simulink model "EF"  (R2023a)
settings: Solver=FixedStepDiscrete  StartTime=0.0  StopTime=inf  FixedStep=50e-6  RelTol=1e-3  EnableMultiTasking=on
libraries: spsThreePhaseFaultLib x11, spsThreePhaseSourceLib x3, spsCurrentMeasurementLib x2, spsDistributedParametersLineLib x2, spsGroundLib x2, spsThreePhaseParallelRLCLoadLib x2, spsThreePhaseTransformer12TerminalsLib x2, spsThreePhaseSeriesRLCLoadLib x1, spsThreePhaseVIMeasurementLib x1, instrumentlib x1, spspowerguiLib x1
settings Model: Creator=Administrator  LastModifiedBy=Ansoufeh
settings SolverCC: AlgebraicLoopSolver=TrustRegion
settings DataIOCC: LimitDataPoints=on  SaveFormat=Array  SignalLoggingSaveFormat=ModelDataLogs  ReturnWorkspaceOutputs=off
settings OptimizationCC: ExpressionDepthLimit=2147483647  LifeSpan=inf
settings DebuggingCC: UnderspecifiedInitializationDetection=Classic  MergeDetectMultiDrivingBlocksExec=none  SolverPrmCheckMsg=warning  FcnCallInpInsideContextMsg=warning  StateNameClashWarn=warning  SFUnexpectedBacktrackingDiag=warning  SFNoUnconditionalDefaultTransitionDiag=warning  SFExecutionAtInitializationDiag=none  ArithmeticOperatorsInVariantConditions=warning
settings HardwareCC: ProdBitPerPointer=32  ProdBitPerSizeT=32  ProdBitPerPtrDiffT=32  ProdLargestAtomicFloat=None  ProdIntDivRoundTo=Undefined  ProdEndianess=Unspecified  ProdWordSize=32  ProdHWDeviceType=32-bit Generic
settings ModelReferenceCC: EnableRefExpFcnMdlSchedulingChecks=on  PropagateSignalLabelsOutOfModel=off
settings SFSimCC: SimUseLocalCustomCode=off  CustomCodeUndefinedFunction=UseInterfaceOnly
settings RTWCC: RTWUseLocalCustomCode=off
settings CodeAppCC: StateflowObjectComments=on
settings GRTTargetCC: TargetLangStandard=C89/C90 (ANSI)  CombineOutputUpdateFcns=off  GRTInterface=on
settings ConfigComp: CovMetricSettings=dw  CovSaveCumulativeToWorkspaceVar=on  CovSaveSingleToWorkspaceVar=on  CovExternalEMLEnable=off  CovSFcnEnable=off
settings SimscapeCC: SimscapeNormalizeSystem=off

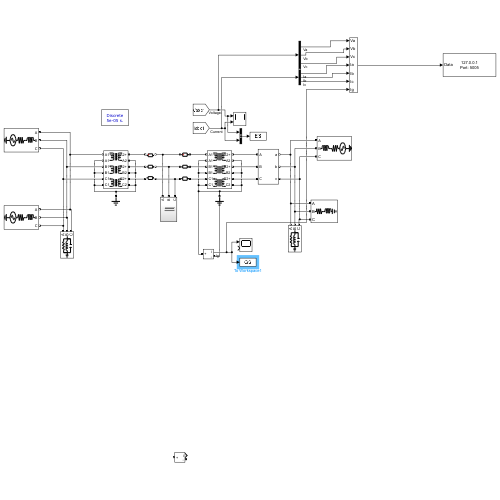
[thumbnail: Simulink's stored preview of the top-level diagram]
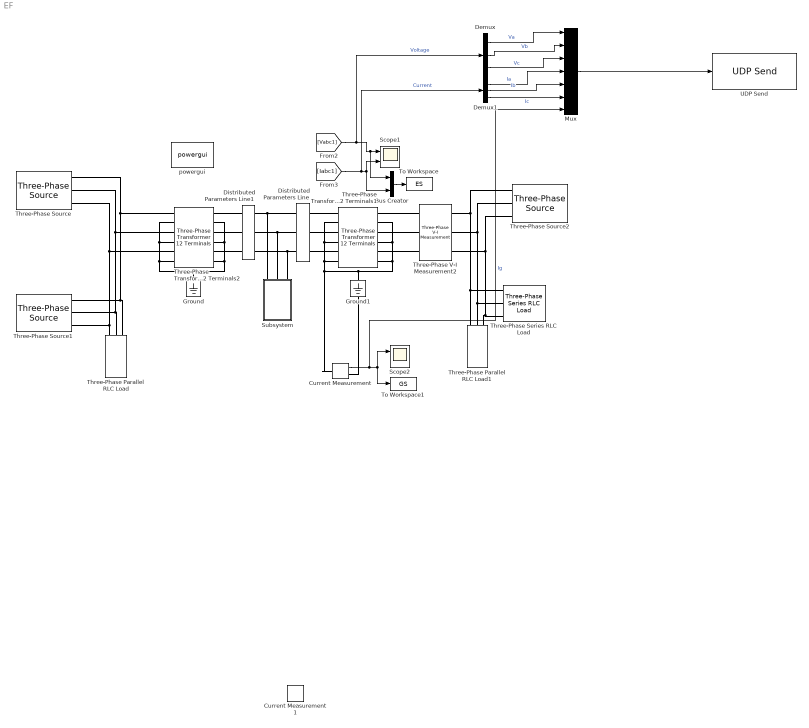
== system EF ==
  Bus Creator : BusCreator  Inputs=2
  Current Measurement : spsCurrentMeasurementLib/Current Measurement  PhasorSimulation=off  OutputType=Complex  PSBequivalent=0
  Current Measurement1 : spsCurrentMeasurementLib/Current Measurement  PhasorSimulation=off  OutputType=Complex  PSBequivalent=0
  Demux : Demux  Outputs=3
  Demux1 : Demux  Outputs=3
  Distributed Parameters Line : spsDistributedParametersLineLib/Distributed Parameters Line  Phases=3  Length=33  Frequency=50  Resistance=[0.0132 0.132]  Inductance="[0.9337e-3  4.1264e-3]"  Capacitance=[12.74e-9 7.751e-9]  x1=[-0.0002 -26194.4990565152 0 0;-0.00015 -25142.4200654069 -14084.2021249757 -139676.156535357;-0.0001 -24084.1375583615 -10869.3978359019 -138608.787184405;-5e-05 -23019.9126507524 -7651.91168555439 -137507.218189264]  x2=[-0.0002 -26508.8832650109 0 0;-0.00015 -25460.9682547841 -14346.2347519264 -139705.26954599;-0.0001 -24406.7711316212 -11133.032561043 -138641.209662973;-5e-05 -23346.5520028879 -7917.08346096219 -137542.942136005]  x3=[-0.0002 -32.9787723954412 0 0;-0.00015 -31.6839639948928 -55.9550231746791 -498.136583373614;-0.0001 -30.3813380503261 -44.5400586108173 -494.408000929939;-5e-05 -29.0712159652011 -33.1141044539605 -490.557430710021]  x4=[-0.0002 -44.2714402477354 0 0;-0.00015 -42.7334839975939 -75.9286566808512 -541.426288335773;-0.0001 -41.1849838997108 -63.6542106681894 -537.579668417394;-5e-05 -39.6263220233146 -51.3640589315235 -533.600408759809]  x5=0.000186628717108595  V1=[2.547e-09 1.32e+05 1.32e+05;314.2 314.2 314.2;-0.1043 0.8095 -0.7613]  V2=[2.522e-09 1.32e+05 1.32e+05;314.2 314.2 314.2;-0.1193 0.8007 -0.7701]  I1=[2.615e-12 367.2 367.2;314.2 314.2 314.2;-0.5343 0.7771 -0.7937]  I2=[5.144e-12 607 607;314.2 314.2 314.2;-0.488 0.7934 -0.7774]  nHarmo=1  Measurements=None  Decoupling=off  VsMag0=0  VrMag0=0  VsAngle0=0  VrAngle0=0  IsMag0=0  IrMag0=0  IsAngle0=0  IrAngle0=0
      settings: LibrarySourceBlock=sps_lib/Power Grid Elements/Distributed Parameters Line
  Distributed Parameters Line1 : spsDistributedParametersLineLib/Distributed Parameters Line  Phases=3  Length=33  Frequency=50  Resistance=[0.0132 0.132]  Inductance="[0.9337e-3  4.1264e-3]"  Capacitance=[12.74e-9 7.751e-9]  x1=[-0.0002 -25744.8060541232 0 0;-0.00015 -24691.8631075608 -13770.6890303449 -139458.191007;-0.0001 -23632.8278132488 -10558.3448334587 -138388.513170059;-5e-05 -22567.9614722995 -7343.39552297271 -137284.690038246]  x2=[-0.0002 -26194.4990565152 0 0;-0.00015 -25142.4200654069 -14084.2021249757 -139676.156535357;-0.0001 -24084.1375583615 -10869.3978359019 -138608.787184405;-5e-05 -23019.9126507524 -7651.91168555439 -137507.218189264]  x3=[-0.0002 -37.5098312649845 0 0;-0.00015 -36.2542690466918 -81.6323668107199 -504.631077447372;-0.0001 -34.989761629996 -70.2873602270549 -501.193965481607;-5e-05 -33.7166210131811 -58.9250112889862 -497.633191404385]  x4=[-0.0002 -38.7109249659307 0 0;-0.00015 -37.1263797926598 -48.124582446735 -534.043951803313;-0.0001 -35.5326742407089 -35.7827477551342 -529.884875428009;-5e-05 -33.930201533076 -23.4320842059535 -525.595057888531]  x5=0.000186628717108595  V1=[2.618e-09 1.319e+05 1.319e+05;314.2 314.2 314.2;-0.1003 0.8184 -0.7524]  V2=[2.549e-09 1.32e+05 1.32e+05;314.2 314.2 314.2;-0.1043 0.8095 -0.7613]  I1=[2.387e-12 367.3 367.3;314.2 314.2 314.2;0.1434 0.7414 -0.8294]  I2=[6.175e-12 607.4 607.4;314.2 314.2 314.2;-0.4569 0.8292 -0.7416]  nHarmo=1  Measurements=None  Decoupling=off  VsMag0=0  VrMag0=0  VsAngle0=0  VrAngle0=0  IsMag0=0  IrMag0=0  IsAngle0=0  IrAngle0=0
      settings: LibrarySourceBlock=sps_lib/Power Grid Elements/Distributed Parameters Line
  Ground : spsGroundLib/Ground  LConnTagsString=a
  Ground1 : spsGroundLib/Ground  LConnTagsString=a
  Mux : Mux  Inputs=7
      settings: DisplayOption=signals
  Scope1 : Scope  NumInputPorts=2
  Scope2 : Scope  NumInputPorts=2
  Subsystem : Subsystem
  Three-Phase Parallel RLC Load : spsThreePhaseParallelRLCLoadLib/Three-Phase Parallel RLC Load  LConnTagsString=A|B|C  Configuration=Y (grounded)  NominalVoltage=1000  Vabc=[1e3 1e3 1e3]  Vabcp=[1e3 1e3 1e3]  NominalFrequency=60  UnbalancedPower=off  ActivePower=10e4  InductivePower=100  CapacitivePower=100  Pabc=[10e3 9e3 11e3]  QLabc=[100 90 110]  QCabc=[100 90 110]  Pabcp=[10e3 9e3 11e3]  QLabcp=[100 90 110]  QCabcp=[100 90 110]  Measurements=None  LoadType=constant Z
  Three-Phase Parallel RLC Load1 : spsThreePhaseParallelRLCLoadLib/Three-Phase Parallel RLC Load  LConnTagsString=A|B|C  Configuration=Y (grounded)  NominalVoltage=1000  Vabc=[1e3 1e3 1e3]  Vabcp=[1e3 1e3 1e3]  NominalFrequency=60  UnbalancedPower=off  ActivePower=100  InductivePower=10  CapacitivePower=10  Pabc=[10e3 9e3 11e3]  QLabc=[100 90 110]  QCabc=[100 90 110]  Pabcp=[10e3 9e3 11e3]  QLabcp=[100 90 110]  QCabcp=[100 90 110]  Measurements=None  LoadType=constant Z
  Three-Phase Series RLC Load : spsThreePhaseSeriesRLCLoadLib/Three-Phase Series RLC Load  LConnTagsString=A|B|C  Configuration=Y (grounded)  NominalVoltage=11e3  Vabc=[1e3 1e3 1e3]  Vabcp=[1e3 1e3 1e3]  NominalFrequency=50  UnbalancedPower=off  ActivePower=10e6  InductivePower=100  CapacitivePower=0  Pabc=[10e3 9e3 11e3]  QLabc=[100 90 110]  QCabc=[100 90 110]  Pabcp=[10e3 9e3 11e3]  QLabcp=[100 90 110]  QCabcp=[100 90 110]  Measurements=None  LoadType=constant Z
  Three-Phase V-I Measurement2 : spsThreePhaseVIMeasurementLib/Three-Phase V-I Measurement  VoltageMeasurement=phase-to-phase  SetLabelV=on  LabelV=Vabc1  Vpu=off  VpuLL=on  CurrentMeasurement=yes  SetLabelI=on  LabelI=Iabc1  Ipu=off  Pbase=100e6  Vbase=11e3  OutputType=Complex  PhasorSimulation=off  PSBequivalent=0
  Three-Phase Source : spsThreePhaseSourceLib/Three-Phase Source  InternalConnection=Yg  VoltagePhases=on  Voltage=11e3  PhaseAngle=0  Voltage_phases=[25e3 11e3 11e3]/sqrt(3)  PhaseAngles_phases=[0 -120 +120]  Frequency=50  NonIdealSource=on  SpecifyImpedance=off  Resistance=1.5  Inductance=16.58e-3  ShortCircuitLevel=50e6  BaseVoltage=11e3  XRratio=7  BusType=PV  Pref=50e6  Qref=0  Prefabc=[10e3, 10e3, 10e3]  Qrefabc=[0, 0, 0]  Qmin=-inf  Qmax=inf
  Three-Phase Source1 : spsThreePhaseSourceLib/Three-Phase Source  InternalConnection=Yg  VoltagePhases=on  Voltage=11e3  PhaseAngle=0  Voltage_phases=[25e3 11e3 11e3]/sqrt(3)  PhaseAngles_phases=[0 -120 +120]  Frequency=50  NonIdealSource=on  SpecifyImpedance=off  Resistance=1.5  Inductance=16.58e-3  ShortCircuitLevel=50e6  BaseVoltage=11e3  XRratio=7  BusType=PV  Pref=50e6  Qref=0  Prefabc=[10e3, 10e3, 10e3]  Qrefabc=[0, 0, 0]  Qmin=-inf  Qmax=inf
  Three-Phase Source2 : spsThreePhaseSourceLib/Three-Phase Source  InternalConnection=Yg  VoltagePhases=on  Voltage=11e3  PhaseAngle=0  Voltage_phases=[25e3 11e3 11e3]/sqrt(3)  PhaseAngles_phases=[0 -120 +120]  Frequency=50  NonIdealSource=on  SpecifyImpedance=off  Resistance=1.5  Inductance=16.58e-3  ShortCircuitLevel=20e6  BaseVoltage=11e3  XRratio=7  BusType=PV  Pref=20e6  Qref=0  Prefabc=[10e3, 10e3, 10e3]  Qrefabc=[0, 0, 0]  Qmin=-inf  Qmax=inf
  Three-Phase Transformer 12 Terminals1 : spsThreePhaseTransformer12TerminalsLib/Three-Phase Transformer 12 Terminals  RatedPower=[100e6 50]  Winding1="[ 132e3 0.002  0.05 ]"  Winding2=[ 11e3 0.002 0.05]  RmXm=[ 200 200 ]
      settings: LibrarySourceBlock=|
      | sps_lib/Power Grid Elements/Three-Phase Transformer
      | 12 Terminals
  Three-Phase Transformer 12 Terminals2 : spsThreePhaseTransformer12TerminalsLib/Three-Phase Transformer 12 Terminals  RatedPower=[100e6 50]  Winding1="[ 11e3 0.002  0.05 ]"  Winding2=[ 132e3 0.002 0.05]  RmXm=[ 200 200 ]
      settings: LibrarySourceBlock=|
      | sps_lib/Power Grid Elements/Three-Phase Transformer
      | 12 Terminals
  To Workspace : ToWorkspace  VariableName=ES  SaveFormat=Structure With Time  SampleTime=-1
  To Workspace1 : ToWorkspace  VariableName=GS  SaveFormat=Structure With Time  SampleTime=-1
  UDP Send : instrumentlib/UDP Send  Host=127.0.0.1  Port=5005  LocalAddress=0.0.0.0  LocalPort=5005  EnablePortSharing=on  OutputDatagramPacketSize=1024  ByteOrder=big-endian  EnableBlockingMode=on  SimulateUsing=Interpreted execution
  powergui : spspowerguiLib/powergui  Priority=1  SimulationMode=Discrete  SampleTime=50e-6  frequency=50  Iterations=50  frequencyindice=50  Pbase=100e6  ErrMax=1e-4  UnitsV=kV  UnitsW=MW  buscounter=0  FunctionMessages=off  echomessages=off  EnableUseOfTLC=off  CurrentSourceSwitches=off  DisableSnubberDevices=off  DisableRonSwitches=off  DisableVfSwitches=off  DisplayEquations=off  AutomaticDiscreteSolvers=off  SolverType=Tustin  Interpol=off  ExternalGateDelay=off  methode=off  Ts=0  x0status=blocks  SPID=off  SwTol=0  HookPort=off  NonlinearTolerance=1e-4  nMaxIteration=100  ContinueOnMaxIteration=off  RestoreLinks=warning  ResistiveCurrentMeasurement=off  Frange=[0:2:500]  Ylog=off  Xlog=on  ShowGrid=off  save=off  variable=ZData  structure=0  ZoomFFT=off  StartTime=0.0  cycles=1  DisplayStyle=1  fundamental=60  FreqAxis=off  MaxFrequency=1000  frequencyindicesteady=1  RmsSteady=1  display=off
  wires:
  [Vabc1] -> Demux/1, Bus Creator/1, Scope1/1  "Voltage"
  [Iabc1] -> Demux1/1, Bus Creator/2, Scope1/2  "Current"
  Bus Creator/1 -> To Workspace/1
  Current Measurement/1 -> Mux/7, To Workspace1/1, Scope2/1  "Ig"
  Demux/1 -> Mux/1  "Va"
  Demux/2 -> Mux/2  "Vb"
  Demux/3 -> Mux/3  "Vc"
  Demux1/1 -> Mux/4  "Ia"
  Demux1/2 -> Mux/5  "Ib"
  Demux1/3 -> Mux/6  "Ic"
  Mux/1 -> UDP Send/1
  connections:
  Distributed Parameters Line1/RConn1 -- Subsystem/LConn1 -- Distributed Parameters Line/LConn1
  Three-Phase Series RLC Load/LConn2 -- Three-Phase Parallel RLC Load1/LConn2 -- Three-Phase V-I Measurement2/RConn2 -- Three-Phase Source2/RConn2
  Distributed Parameters Line1/RConn3 -- Subsystem/LConn3 -- Distributed Parameters Line/LConn3
  Three-Phase Series RLC Load/LConn1 -- Three-Phase Parallel RLC Load1/LConn1 -- Three-Phase V-I Measurement2/RConn1 -- Three-Phase Source2/RConn1
  Distributed Parameters Line1/RConn2 -- Subsystem/LConn2 -- Distributed Parameters Line/LConn2
  Three-Phase Series RLC Load/LConn3 -- Three-Phase Parallel RLC Load1/LConn3 -- Three-Phase V-I Measurement2/RConn3 -- Three-Phase Source2/RConn3
  Three-Phase Transformer 12 Terminals2/RConn1 -- Distributed Parameters Line1/LConn1
  Three-Phase Transformer 12 Terminals2/RConn3 -- Distributed Parameters Line1/LConn2
  Three-Phase Transformer 12 Terminals2/RConn5 -- Distributed Parameters Line1/LConn3
  Three-Phase Source/RConn2 -- Three-Phase Transformer 12 Terminals2/LConn3 -- Three-Phase Parallel RLC Load/LConn2 -- Three-Phase Source1/RConn2
  Three-Phase Source/RConn1 -- Three-Phase Transformer 12 Terminals2/LConn1 -- Three-Phase Parallel RLC Load/LConn3 -- Three-Phase Source1/RConn1
  Three-Phase Source/RConn3 -- Three-Phase Transformer 12 Terminals2/LConn5 -- Three-Phase Parallel RLC Load/LConn1 -- Three-Phase Source1/RConn3
  Ground/LConn1 -- Three-Phase Transformer 12 Terminals2/LConn6 -- Three-Phase Transformer 12 Terminals2/LConn4 -- Three-Phase Transformer 12 Terminals2/LConn2 -- Three-Phase Transformer 12 Terminals2/RConn6 -- Three-Phase Transformer 12 Terminals2/RConn4 -- Three-Phase Transformer 12 Terminals2/RConn2
  Ground1/LConn1 -- Current Measurement/LConn1 -- Three-Phase Transformer 12 Terminals1/LConn6 -- Three-Phase Transformer 12 Terminals1/LConn4 -- Three-Phase Transformer 12 Terminals1/LConn2 -- Current Measurement/RConn1 -- Three-Phase Transformer 12 Terminals1/RConn6 -- Three-Phase Transformer 12 Terminals1/RConn4 -- Three-Phase Transformer 12 Terminals1/RConn2
  Three-Phase V-I Measurement2/LConn1 -- Three-Phase Transformer 12 Terminals1/RConn1
  Three-Phase V-I Measurement2/LConn2 -- Three-Phase Transformer 12 Terminals1/RConn3
  Three-Phase V-I Measurement2/LConn3 -- Three-Phase Transformer 12 Terminals1/RConn5
  Distributed Parameters Line/RConn3 -- Three-Phase Transformer 12 Terminals1/LConn5
  Distributed Parameters Line/RConn2 -- Three-Phase Transformer 12 Terminals1/LConn3
  Distributed Parameters Line/RConn1 -- Three-Phase Transformer 12 Terminals1/LConn1

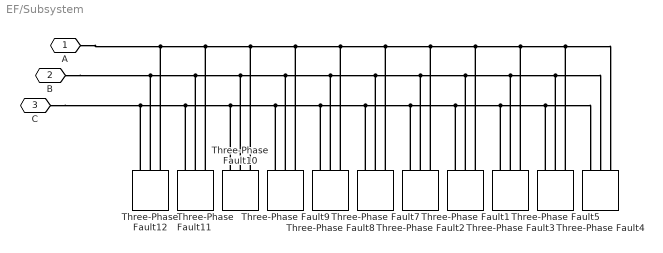
== system EF/Subsystem ==
  Three-Phase Fault1 : spsThreePhaseFaultLib/Three-Phase Fault  InitialStates=0  FaultA=on  FaultB=on  FaultC=off  GroundFault=off  SwitchTimes=[4.650, 5.250]  External=off  SwitchStatus=NaN  FaultResistance=0.001  GroundResistance=0.001  SnubberResistance=1e6  SnubberCapacitance=inf  Measurements=None
  Three-Phase Fault10 : spsThreePhaseFaultLib/Three-Phase Fault  InitialStates=0  FaultA=off  FaultB=on  FaultC=on  GroundFault=off  SwitchTimes=[1.400, 2.000]  External=off  SwitchStatus=NaN  FaultResistance=0.001  GroundResistance=0.001  SnubberResistance=1e6  SnubberCapacitance=inf  Measurements=None
  Three-Phase Fault11 : spsThreePhaseFaultLib/Three-Phase Fault  InitialStates=0  FaultA=on  FaultB=off  FaultC=off  GroundFault=on  SwitchTimes=[0.750, 1.350]  External=off  SwitchStatus=NaN  FaultResistance=0.001  GroundResistance=0.001  SnubberResistance=1e6  SnubberCapacitance=inf  Measurements=None
  Three-Phase Fault12 : spsThreePhaseFaultLib/Three-Phase Fault  InitialStates=0  FaultA=on  FaultB=on  FaultC=off  GroundFault=on  SwitchTimes=[0.100, 0.700]  External=off  SwitchStatus=NaN  FaultResistance=0.001  GroundResistance=0.001  SnubberResistance=1e6  SnubberCapacitance=inf  Measurements=None
  Three-Phase Fault2 : spsThreePhaseFaultLib/Three-Phase Fault  InitialStates=0  FaultA=off  FaultB=off  FaultC=on  GroundFault=on  SwitchTimes=[4.000, 4.600]  External=off  SwitchStatus=NaN  FaultResistance=0.001  GroundResistance=0.001  SnubberResistance=1e6  SnubberCapacitance=inf  Measurements=None
  Three-Phase Fault3 : spsThreePhaseFaultLib/Three-Phase Fault  InitialStates=0  FaultA=on  FaultB=off  FaultC=on  GroundFault=off  SwitchTimes=[5.300, 5.900]  External=off  SwitchStatus=NaN  FaultResistance=0.001  GroundResistance=0.001  SnubberResistance=1e6  SnubberCapacitance=inf  Measurements=None
  Three-Phase Fault4 : spsThreePhaseFaultLib/Three-Phase Fault  InitialStates=0  FaultA=on  FaultB=on  FaultC=on  GroundFault=on  SwitchTimes=[7.200, 8.400]  External=off  SwitchStatus=NaN  FaultResistance=0.001  GroundResistance=0.001  SnubberResistance=1e6  SnubberCapacitance=inf  Measurements=None
  Three-Phase Fault5 : spsThreePhaseFaultLib/Three-Phase Fault  InitialStates=0  FaultA=on  FaultB=on  FaultC=on  GroundFault=off  SwitchTimes=[5.950, 7.150]  External=off  SwitchStatus=NaN  FaultResistance=0.001  GroundResistance=0.001  SnubberResistance=1e6  SnubberCapacitance=inf  Measurements=None
  Three-Phase Fault7 : spsThreePhaseFaultLib/Three-Phase Fault  InitialStates=0  FaultA=off  FaultB=on  FaultC=off  GroundFault=on  SwitchTimes=[3.350, 3.950]  External=off  SwitchStatus=NaN  FaultResistance=0.001  GroundResistance=0.001  SnubberResistance=1e6  SnubberCapacitance=inf  Measurements=None
  Three-Phase Fault8 : spsThreePhaseFaultLib/Three-Phase Fault  InitialStates=0  FaultA=off  FaultB=on  FaultC=on  GroundFault=on  SwitchTimes=[2.700, 3.300]  External=off  SwitchStatus=NaN  FaultResistance=0.001  GroundResistance=0.001  SnubberResistance=1e6  SnubberCapacitance=inf  Measurements=None
  Three-Phase Fault9 : spsThreePhaseFaultLib/Three-Phase Fault  InitialStates=0  FaultA=on  FaultB=off  FaultC=on  GroundFault=on  SwitchTimes=[2.050, 2.650]  External=off  SwitchStatus=NaN  FaultResistance=0.001  GroundResistance=0.001  SnubberResistance=1e6  SnubberCapacitance=inf  Measurements=None
  A : PMIOPort  Side=Left
  B : PMIOPort  Port=2  Side=Left
  C : PMIOPort  Port=3  Side=Left
  connections:
  A/RConn1 -- Three-Phase Fault11/LConn1 -- Three-Phase Fault9/LConn1 -- Three-Phase Fault8/LConn1 -- Three-Phase Fault7/LConn1 -- Three-Phase Fault2/LConn1 -- Three-Phase Fault1/LConn1 -- Three-Phase Fault3/LConn1 -- Three-Phase Fault5/LConn1 -- Three-Phase Fault4/LConn1 -- Three-Phase Fault10/LConn1 -- Three-Phase Fault12/LConn1
  B/RConn1 -- Three-Phase Fault12/LConn2 -- Three-Phase Fault11/LConn2 -- Three-Phase Fault10/LConn2 -- Three-Phase Fault9/LConn2 -- Three-Phase Fault8/LConn2 -- Three-Phase Fault7/LConn2 -- Three-Phase Fault2/LConn2 -- Three-Phase Fault1/LConn2 -- Three-Phase Fault3/LConn2 -- Three-Phase Fault5/LConn2 -- Three-Phase Fault4/LConn2
  C/RConn1 -- Three-Phase Fault12/LConn3 -- Three-Phase Fault11/LConn3 -- Three-Phase Fault10/LConn3 -- Three-Phase Fault9/LConn3 -- Three-Phase Fault8/LConn3 -- Three-Phase Fault7/LConn3 -- Three-Phase Fault2/LConn3 -- Three-Phase Fault1/LConn3 -- Three-Phase Fault3/LConn3 -- Three-Phase Fault5/LConn3 -- Three-Phase Fault4/LConn3
